simulink model "simulink_03"  (R2021a)
settings: Solver=VariableStepAuto  StartTime=0.0  StopTime=48  RelTol=1e-3
settings Model: Creator=alamg  LastModifiedBy=alamg

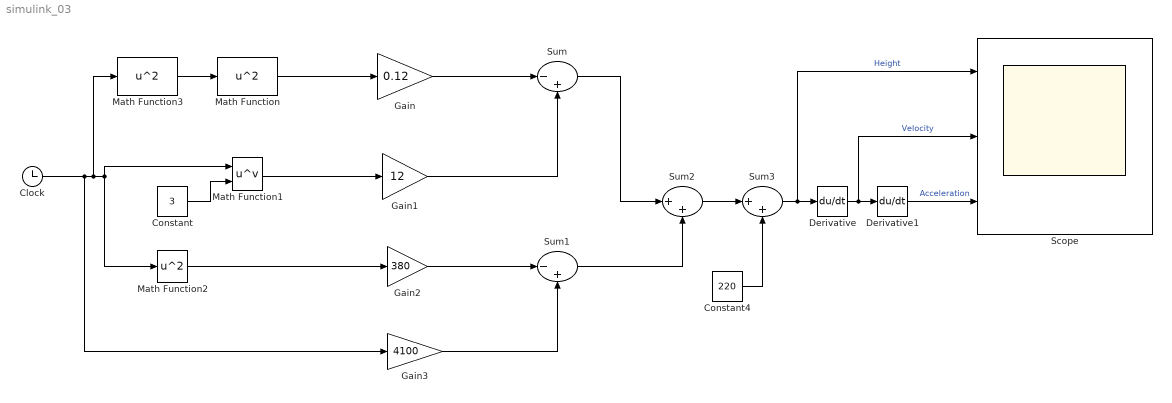
== system simulink_03 ==
  Clock : Clock
  Constant : Constant  Value=3
  Constant4 : Constant  Value=220
  Derivative : Derivative
  Derivative1 : Derivative
  Gain : Gain  Gain=0.12
  Gain1 : Gain  Gain=12
  Gain2 : Gain  Gain=380
  Gain3 : Gain  Gain=4100
  Math Function : Math  Operator=square  SaturateOnIntegerOverflow=on
  Math Function1 : Math  Operator=pow  SaturateOnIntegerOverflow=on
  Math Function2 : Math  Operator=square  SaturateOnIntegerOverflow=on
  Math Function3 : Math  Operator=square  SaturateOnIntegerOverflow=on
  Scope : Scope  NumInputPorts=3
  Sum : Sum  Inputs=|-+
  Sum1 : Sum  Inputs=|-+
  Sum2 : Sum  Inputs=|++
  Sum3 : Sum  Inputs=|++
  wires:
  Derivative1/1 -> Scope/3  "Acceleration"
  Gain/1 -> Sum/1
  Gain1/1 -> Sum/2
  Gain2/1 -> Sum1/1
  Gain3/1 -> Sum1/2
  Sum/1 -> Sum2/1
  Sum1/1 -> Sum2/2
  Clock/1 -> Gain3/1, Math Function1/1, Math Function2/1, Math Function3/1
  Math Function2/1 -> Gain2/1
  Math Function1/1 -> Gain1/1
  Math Function/1 -> Gain/1
  Sum3/1 -> Scope/1, Derivative/1  "Height"
  Sum2/1 -> Sum3/1
  Constant4/1 -> Sum3/2
  Derivative/1 -> Scope/2, Derivative1/1  "Velocity"
  Math Function3/1 -> Math Function/1
  Constant/1 -> Math Function1/2
